simulink model "task_32_sim"  (R2023a)
settings: Solver=VariableStepAuto  StartTime=0.0  StopTime=8  MaxStep=1e-4  RelTol=1e-4
undefined symbols (not defined in the file): A, B, Bf, C, D, Df, G, G_f, G_g, Gf2, iQ, iQf, K, Kf, Kg, w_f0, w_g0, x0, Y, Y_f, Y_g, Yf2
settings Model: Creator=user  LastModifiedBy=user

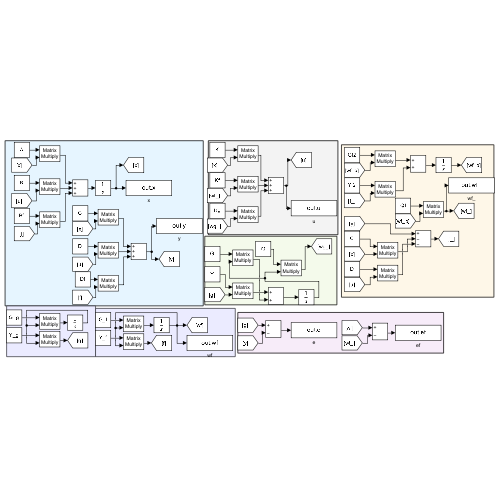
[thumbnail: Simulink's stored preview of the top-level diagram]
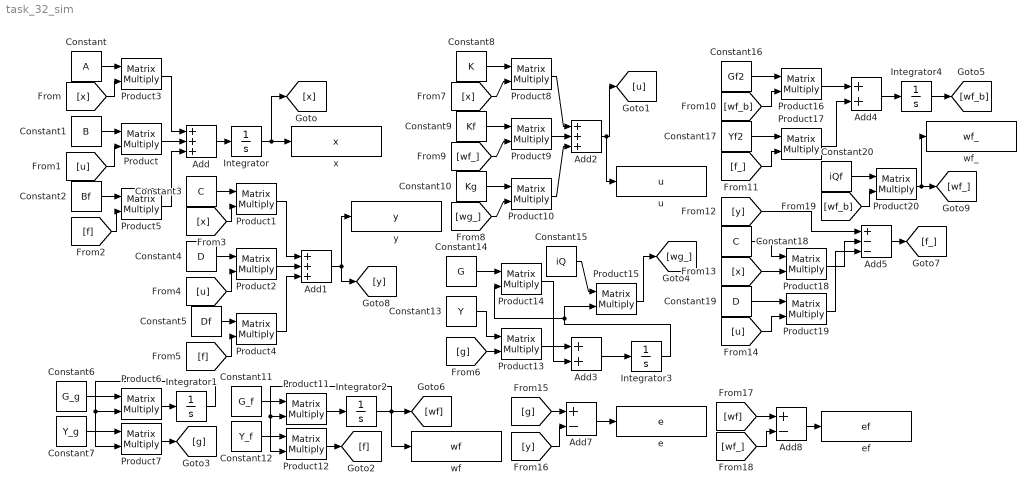
== system task_32_sim ==
  Add : Sum  Inputs=+++
  Add1 : Sum  Inputs=+++
  Add2 : Sum  Inputs=+++
  Add3 : Sum
  Add4 : Sum
  Add5 : Sum  Inputs=+--
  Add7 : Sum  Inputs=+-
  Add8 : Sum  Inputs=+-
  Constant : Constant  Value=A  VectorParams1D=off
  Constant1 : Constant  Value=B  VectorParams1D=off
  Constant10 : Constant  Value=Kg  VectorParams1D=off
  Constant11 : Constant  Value=G_f  VectorParams1D=off
  Constant12 : Constant  Value=Y_f  VectorParams1D=off
  Constant13 : Constant  Value=Y  VectorParams1D=off
  Constant14 : Constant  Value=G  VectorParams1D=off
  Constant15 : Constant  Value=iQ  VectorParams1D=off
  Constant16 : Constant  Value=Gf2  VectorParams1D=off
  Constant17 : Constant  Value=Yf2  VectorParams1D=off
  Constant18 : Constant  Value=C  VectorParams1D=off
  Constant19 : Constant  Value=D  VectorParams1D=off
  Constant2 : Constant  Value=Bf  VectorParams1D=off
  Constant20 : Constant  Value=iQf  VectorParams1D=off
  Constant3 : Constant  Value=C  VectorParams1D=off
  Constant4 : Constant  Value=D  VectorParams1D=off
  Constant5 : Constant  Value=Df  VectorParams1D=off
  Constant6 : Constant  Value=G_g  VectorParams1D=off
  Constant7 : Constant  Value=Y_g  VectorParams1D=off
  Constant8 : Constant  Value=K  VectorParams1D=off
  Constant9 : Constant  Value=Kf  VectorParams1D=off
  Integrator : Integrator  InitialCondition=x0
  Integrator1 : Integrator  InitialCondition=w_g0
  Integrator2 : Integrator  InitialCondition=w_f0
  Integrator3 : Integrator
  Integrator4 : Integrator
  Product{,1..20} (21 alike) : Product  Multiplication=Matrix(*)
  e : ToWorkspace  VariableName=e  SaveFormat=Timeseries  SampleTime=-1
  ef : ToWorkspace  VariableName=ef  SaveFormat=Timeseries  SampleTime=-1
  u : ToWorkspace  VariableName=u  SaveFormat=Timeseries  SampleTime=-1
  wf : ToWorkspace  VariableName=wf  SaveFormat=Timeseries  SampleTime=-1
  wf_ : ToWorkspace  VariableName=wf_  SaveFormat=Timeseries  SampleTime=-1
  x : ToWorkspace  VariableName=x  SaveFormat=Timeseries  SampleTime=-1
  y : ToWorkspace  VariableName=y  SaveFormat=Timeseries  SampleTime=-1
  wires:
  Constant/1 -> Product3/1
  Constant1/1 -> Product/1
  Constant2/1 -> Product5/1
  [x] -> Product3/2
  [u] -> Product/2
  [f] -> Product5/2
  Constant3/1 -> Product1/1
  [x] -> Product1/2
  Constant4/1 -> Product2/1
  [u] -> Product2/2
  Constant5/1 -> Product4/1
  [f] -> Product4/2
  Product/1 -> Add/2
  Product3/1 -> Add/1
  Product5/1 -> Add/3
  Product2/1 -> Add1/2
  Product1/1 -> Add1/1
  Product4/1 -> Add1/3
  Add/1 -> Integrator/1
  Integrator/1 -> [x], x/1
  Add1/1 -> y/1, [y]
  Integrator1/1 -> Product6/2, Product7/2
  Constant6/1 -> Product6/1
  Product6/1 -> Integrator1/1
  Constant7/1 -> Product7/1
  Product7/1 -> [g]
  Constant8/1 -> Product8/1
  [x] -> Product8/2
  Constant9/1 -> Product9/1
  [wf_] -> Product9/2
  Constant10/1 -> Product10/1
  [wg_] -> Product10/2
  Product9/1 -> Add2/2
  Product8/1 -> Add2/1
  Product10/1 -> Add2/3
  Add2/1 -> [u], u/1
  Constant11/1 -> Product11/1
  Product12/1 -> [f]
  Integrator2/1 -> [wf], wf/1, Product11/2, Product12/2
  Product11/1 -> Integrator2/1
  Constant12/1 -> Product12/1
  Constant13/1 -> Product13/1
  [g] -> Product13/2
  Product13/1 -> Add3/1
  Add3/1 -> Integrator3/1
  Constant14/1 -> Product14/1
  Integrator3/1 -> Product15/2, Product14/2
  Product14/1 -> Add3/2
  Constant15/1 -> Product15/1
  Product15/1 -> [wg_]
  [g] -> Add7/1
  [y] -> Add7/2
  Add7/1 -> e/1
  [wf] -> Add8/1
  [wf_] -> Add8/2
  Add8/1 -> ef/1
  Constant16/1 -> Product16/1
  [wf_b] -> Product16/2
  Constant17/1 -> Product17/1
  [f_] -> Product17/2
  Product16/1 -> Add4/1
  Product17/1 -> Add4/2
  Add4/1 -> Integrator4/1
  Integrator4/1 -> [wf_b]
  Constant19/1 -> Product19/1
  [u] -> Product19/2
  [x] -> Product18/2
  Constant18/1 -> Product18/1
  [y] -> Add5/1
  Product18/1 -> Add5/2
  Product19/1 -> Add5/3
  Add5/1 -> [f_]
  Product20/1 -> wf_/1, [wf_]
  Constant20/1 -> Product20/1
  [wf_b] -> Product20/2
